simulink model "windEmulatorStep4_WECSim"  (R2025b)
settings: Solver=ode14x  StartTime=0  StopTime=400  FixedStep=Ts  MaxStep=0.01  RelTol=1e-3
values from neighbouring files (symbols this model uses):
  A = 1.0    (= 1)    [initStep4.m]
  absEncoderCountsToRad = 1/2^20*2*pi    (= 5.99211245268e-06)    [initStep4.m]
  acs800CtrlStruct =     [windEmulatorBusDefs.mat]
  acs800DcBusVoltsScaling = 1    [initStep4.m]
  acs800FreqScaling = 1/100    (= 0.01)    [initStep4.m]
  acs800PowerScaling = Gen_PowerScaling    (= 14.9109)    [initStep4.m]
  acs800SignalStruct =     [windEmulatorBusDefs.mat]
  acs800SpeedNomEng = 1500    [initStep4.m]
  acs800SpeedNomFb = 20000    [initStep4.m]
  acs800SpeedScaling = 1500/20000    (= 0.075)    [initStep4.m]
  acs800TempScaling = 1/10    (= 0.1)    [initStep4.m]
  acs800TorqueNomEng = 100    [initStep4.m]
  acs800TorqueNomFb = 10000    [initStep4.m]
  acs800TorqueScaling = acs800TorqueRating/10000    (= 0.008035933)    [initStep4.m]
  acs880CtrlStruct =     [windEmulatorBusDefs.mat]
  acs880FreqScaling = 60/20000    (= 0.003)    [initStep4.m]
  acs880MotorCurrentScaling = 100/10000    (= 0.01)    [initStep4.m]
  acs880MotorVoltsScaling = 1    [initStep4.m]
  acs880PowerScaling = 100*hp2W/10000    (= 7.457)    [initStep4.m]
  acs880RatedTorque = 80.494    [initStep4.m]
  acs880RateLimFalling = -10000    [initStep4.m]
  acs880RateLimRising = 10000    [initStep4.m]
  acs880SetpointLimLower = -0.975*acs880RatedTorque    (= -78.48165)    [initStep4.m]
  acs880SetpointLimUpper = 0.975*acs880RatedTorque    (= 78.48165)    [initStep4.m]
  acs880SignalStruct =     [windEmulatorBusDefs.mat]
  acs880SpeedPILimLo = -0.975*acs880RatedTorque    (= -78.48165)    [initStep4.m]
  acs880SpeedPILimUp = 0.975*acs880RatedTorque    (= 78.48165)    [initStep4.m]
  acs880SpeedScaling = 2000/20000    (= 0.1)    [initStep4.m]
  acs880TorqueFieldbusScale = 10000    [initStep4.m]
  acs880TorqueScaling = acs880RatedTorque/acs880TorqueFieldbusScale    (= 0.0080494)    [initStep4.m]
  acs880TorqueSetpointScaling = 100    [initStep4.m]
  bar2pa = 1e5    (= 100000)    [initStep4.m]
  belowMinPGain = 1/200    (= 0.005)    [initStep4.m]
  ctrlModeTorque = logical(true)    [init.m]    (also in initStep1.m; initStep2.m; initStep3.m; initStep4.m)
  ctrlSignal1 = squeeze(hptoSignalsData.Values.ctrlSignal1.Data)    [postProcessingStep2.m]
  ctrlSignal2 = squeeze(hptoSignalsData.Values.ctrlSignal2.Data)    [postProcessingStep2.m]
  deadBandController = boolean(false)    [initStep4.m]
  deadbandTorqueSlewRate = 300    [initStep4.m]
  Dm_max = 40    [initStep4.m]
  EffMechMax = 0.93    [initStep4.m]
  EffMechMin = 0.79    [initStep4.m]
  excForce_N = squeeze(hptoCtrlData.Values.excForce_N.Data)    [postProcessingStep2.m]
  expCtrlStruct =     [windEmulatorBusDefs.mat]
  FactorEff = psi2pa*cc2m3*(1/rev2rad)    (= 0.00109733470463)    [initStep4.m]
  fromFileSpeedSlewRate = 250    [initStep4.m]
  fromFileTorqueSlewRate = 25    [initStep4.m]
  futekTorqueScale = -1/(2^31)*10/5*100    (= -9.31322574615e-08)    [initStep4.m]
  genMaxTorque = 0.8*ratedTorque    (= 64.3952)    [initStep3.m]    (also in initStep4.m = 78.48165)
  genTorqueCmd_Nm = squeeze(hptoSignalsData.Values.genTorqueCmd_Nm.Data)    [postProcessingStep2.m]
  hbmCtScale = 1/1.5    (= 0.666666666667)    [initStep4.m]
  hbmPowerStruct =     [windEmulatorBusDefs.mat]
  hptoCtrlStruct =     [windEmulatorBusDefs.mat]
  hptoSignalStruct =     [windEmulatorBusDefs.mat]
  invPowerStruct =     [windEmulatorBusDefs.mat]
  lpm2m3ps = 1/m3ps2lpm    (= 1.66666666667e-05)    [initStep4.m]
  minPressureRef_psi = 1000    [initStep4.m]
  minTorqueRef_Nm = (minPressureRef_psi*psi2pa)*(Dm_max*cc2m3*(1/rev2rad))    (= 43.8933881851)    [initStep4.m]
  motorSpeed_rpm = squeeze(acs880SignalsData.Values.motorSpeed_rpm.Data)    [postProcessingStep2.m]
  nPreDrop = 2900    [initStep4.m]
  nPreDropMin = 725    [initStep4.m]
  psi2bar = 1/bar2psi    (= 0.0689475729318)    [initStep4.m]
  radps2rpm = 60/(2*pi)    (= 9.54929658551)    [initStep2.m]    (also in initStep4.m)
  rpm2radps = 2*pi/60    (= 0.10471975512)    [initStep4.m]
  runCounter = squeeze(hptoCtrlData.Values.runCounter.Data)    [postProcessingStep2.m]
  shaftSignalStruct =     [windEmulatorBusDefs.mat]
  sidCtrlStruct =     [windEmulatorBusDefs.mat]
  sidDataCaseCounter = sidData.experimentData.count    [initStep4.m]
  sidDataSpeed_rpm = sidData.experimentData.wShaft_rpm    [initStep4.m]
  sidDataTorque_Nm = sidData.experimentData.torqueShaft_Nm    [initStep4.m]
  sidInfoStruct =     [windEmulatorBusDefs.mat]
  T = 4    [initStep4.m]
  targetOmega = 2000/60*2*pi    (= 209.439510239)    [initStep2.m]    (also in initStep3.m; initStep4.m)
  time = hptoCtrlData.Values.runCounter.Time    [postProcessingStep2.m]
  TorqueLoadMax = 75    [initStep4.m]
  Ts = 1/250    (= 0.004)    [initStep4.m]
undefined symbols (not defined in the file or in its folder): absEncoderCounts, absEncoderPosition_rad, absEncoderSpeed_rpm, absEncoderStatus1, absEncoderStatus2, absEncoderTurns, accVolHP, acs800Torque_Nm, acs800TorqueSetpoint_Nm, acs880SpeedSetpoint_rpm, acs880Torque_Nm, body, constraint, crankLength, ctrlWord, dcBusVoltage_V, DiscIntNeverNeededParam, Dmax, excShaftSpeed_rpm, excShaftTorque_Nm, expType, expTypeEnum, frequency_Hz, fromFileCaseCounter, genPumpFlow_lpm, genShaftSpeed_rpm, genShaftSpeedRef, genSpeedActual, hmOutputShafTorque_Nm, iGainGen, m3persecond2lpm, motorCurrent_A, motorTorque_Nm, motorVoltage_V, offsetLength, pa2psi, pGainGen, pressure_bar, PressureControl, pto, radsec2rpm, ramp, resetHilIntegrator, resetSidIntegrator, rodLength, runHil, runSid, shaftPower_W, sidType, sidTypeEnum, SpeedControl, speedCtrlReset, speedRef_rpm, state, statusWord, stepCounter, temperature, torqueActual_Nm, TorqueInputControl, torqueSetpoint_Nm ... (+1)
libraries: slrealtimeethercatlib x118, fl_lib x81, nesl_utility x45, sh_lib x18, slrealtimeloglib x13, dspstat3 x5, slpidlib x4, simulink_extras x4, cstblocks x3, dspindex x3, WECSim_Lib_Body_Elements x2, simulink x2
(part 4 of 6)

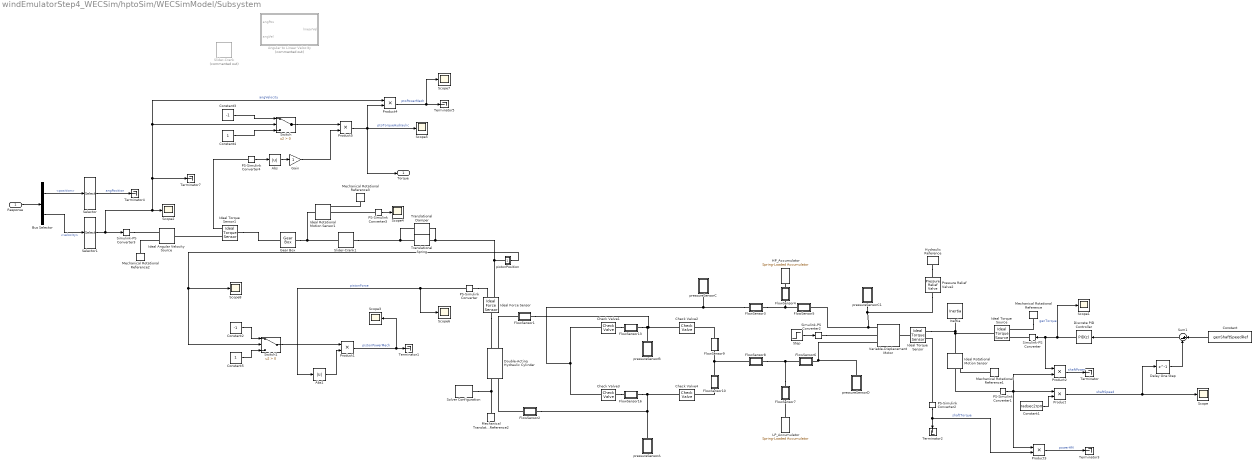
== system windEmulatorStep4_WECSim/hptoSim/WECSimModel/Subsystem ==
  Response : Inport
  Abs : Abs  SaturateOnIntegerOverflow=off
  Abs1 : Abs  SaturateOnIntegerOverflow=off
  Angular to Linear Velocity : Subsystem  Commented=on  AncestorBlock=|
      | WECSim_Lib_PTOSim/Motion Conversion/Rotary to Linear
      | Crank/Angular to Linear
      | Velocity
  Bus Selector : BusSelector  OutputSignals=position,velocity
  Check Valve1 : sh_lib/Valves/Directional Valves/Check Valve  area_max=areaMaxValve m^2  pres_crack=pCrack psi  pres_max=pMaxValve psi  C_d=0.7  A_leak=1e-12 m^2  lam_spec=1  B_lam=0.999  Re_cr=12  dynamic=0  tau=0.1 s  area_init=1e-12 m^2
      settings: InternalSimscapePortConfiguration="{\"Bottom\":[],\"Left\":[{\"id\":\"A\",\"label\":\"A\",\"type\":\"foundation.hydraulic.hydraulic\"}],\"Right\":[{\"id\":\"B\",\"label\":\"B\",\"type\":\"foundation.hydraulic.hydraulic\"}],\"Top\":[]}"
  Check Valve2 : sh_lib/Valves/Directional Valves/Check Valve  area_max=areaMaxValveLP m^2  pres_crack=pCrackLP psi  pres_max=pMaxValveLP psi  C_d=0.7  A_leak=1e-12 m^2  lam_spec=1  B_lam=0.999  Re_cr=12  dynamic=0  tau=0.1 s  area_init=1e-12 m^2
      settings: InternalSimscapePortConfiguration="{\"Bottom\":[],\"Left\":[{\"id\":\"A\",\"label\":\"A\",\"type\":\"foundation.hydraulic.hydraulic\"}],\"Right\":[{\"id\":\"B\",\"label\":\"B\",\"type\":\"foundation.hydraulic.hydraulic\"}],\"Top\":[]}"
  Check Valve3 : sh_lib/Valves/Directional Valves/Check Valve  area_max=areaMaxValve m^2  pres_crack=pCrack psi  pres_max=pMaxValve psi  C_d=0.7  A_leak=1e-12 m^2  lam_spec=1  B_lam=0.999  Re_cr=12  dynamic=0  tau=0.1 s  area_init=1e-12 m^2
      settings: InternalSimscapePortConfiguration="{\"Bottom\":[],\"Left\":[{\"id\":\"A\",\"label\":\"A\",\"type\":\"foundation.hydraulic.hydraulic\"}],\"Right\":[{\"id\":\"B\",\"label\":\"B\",\"type\":\"foundation.hydraulic.hydraulic\"}],\"Top\":[]}"
  Check Valve4 : sh_lib/Valves/Directional Valves/Check Valve  area_max=areaMaxValveLP m^2  pres_crack=pCrackLP psi  pres_max=pMaxValveLP psi  C_d=0.7  A_leak=1e-12 m^2  lam_spec=1  B_lam=0.999  Re_cr=12  dynamic=0  tau=0.1 s  area_init=1e-12 m^2
      settings: InternalSimscapePortConfiguration="{\"Bottom\":[],\"Left\":[{\"id\":\"A\",\"label\":\"A\",\"type\":\"foundation.hydraulic.hydraulic\"}],\"Right\":[{\"id\":\"B\",\"label\":\"B\",\"type\":\"foundation.hydraulic.hydraulic\"}],\"Top\":[]}"
  Constant : Constant  Value=genShaftSpeedRef
  Constant1 : Constant  Value=radsec2rpm
  Constant2 : Constant  Value=-1
  Constant3 : Constant  Value=-1
  Constant4 : Constant
  Constant5 : Constant
  Delay One Step : Delay  DelayLength=1
  Discrete PID Controller : slpidlib/PID Controller  Controller=PID  Form=Parallel  TimeDomain=Discrete-time  UseExternalTs=off  SampleTime=-1  IntegratorMethod=Forward Euler  FilterMethod=Forward Euler  ControllerParametersSource=internal  P=pGainGen  I=iGainGen  UseKiTs=off  D=0  UseExternalDerivativeSource=off  N=100  UseFilter=off  TunerSelectOption=Transfer Function Based (PID Tuner App)  InitialConditionSource=internal  InitialConditionForIntegrator=0  InitialConditionForFilter=0  DifferentiatorICPrevScaledInput=0  ExternalReset=none  TrackingMode=off  Kt=1  LimitOutput=off  SatLimitsSource=internal  UpperSaturationLimit=inf  LowerSaturationLimit=-inf  LinearizeAsGain=off  AntiWindupMode=none  Kb=1  LimitIntegrator=off  UpperIntegratorSaturationLimit=inf  LowerIntegratorSaturationLimit=-inf  POutMin=[]  POutMax=[]  IOutMin=[]  IOutMax=[]  DOutMin=[]  DOutMax=[]  NOutMin=[]  NOutMax=[]  SumOutMin=[]  SumOutMax=[]  SaturationOutMin=[]  SaturationOutMax=[]  PParamMin=[]  PParamMax=[]  IParamMin=[]  IParamMax=[]  DParamMin=[]  DParamMax=[]  NParamMin=[]  NParamMax=[]  KbParamMin=[]  KbParamMax=[]  KtParamMin=[]  KtParamMax=[]  KbOutMin=[]  KbOutMax=[]  KtOutMin=[]  KtOutMax=[]  IntegratorOutMin=[]  IntegratorOutMax=[]  FilterOutMin=[]  FilterOutMax=[]  SumI1OutMin=[]  SumI1OutMax=[]  SumI2OutMin=[]  SumI2OutMax=[]  SumI3OutMin=[]  SumI3OutMax=[]  SumI4OutMin=[]  SumI4OutMax=[]  SumDOutMin=[]  SumDOutMax=[]  DifferentiatorOutMin=[]  DifferentiatorOutMax=[]  FilterDiffOutCoefMin=[]  FilterDiffOutCoefMax=[]  ReciprocalOutMin=[]  ReciprocalOutMax=[]  SumDenOutMin=[]  SumDenOutMax=[]  SumNumOutMin=[]  SumNumOutMax=[]  DivideOutMin=[]  DivideOutMax=[]  UdiffTsProdOutMin=[]  UdiffTsProdOutMax=[]  NTsProdOutMin=[]  NTsProdOutMax=[]  UintegralTsProdOutMin=[]  UintegralTsProdOutMax=[]  UngainTsProdOutMin=[]  UngainTsProdOutMax=[]  ClampingZeroOutDataTypeStr=Inherit: Inherit via back propagation  ClampingZeroOutMin=[]  ClampingZeroOutMax=[]  FilterDenConstantOutDataTypeStr=Inherit: Inherit via back propagation  FilterDenConstantOutMin=[]  FilterDenConstantOutMax=[]  PCopyOutDataTypeStr=Inherit: Inherit via back propagation  PCopyOutMin=[]  PCopyOutMax=[]  NCopyOutDataTypeStr=Inherit: Inherit via back propagation  NCopyOutMin=[]  NCopyOutMax=[]  IntegratorContinuousStateAttributes=''  IntegratorStateMustResolveToSignalObject=off  IntegratorRTWStateStorageClass=Auto  FilterContinuousStateAttributes=''  FilterStateMustResolveToSignalObject=off  FilterRTWStateStorageClass=Auto  ParallelPVariant=InternalParameters  IdealPVariant=Disabled  IVariant=InternalParameters  DVariant=InternalParameters  IntegratorVariant=Discrete  SatVariant=Disabled  AWVariant=Passthrough  PCopyVariant=Disabled  TRVariant=Disabled  FdbkBlocksVariant=Forward  IdealPFdbkVariant=Disabled  SatFdbkVariant=Disabled  DerivativeFilterVariant=Differentiator  NVariant=Passthrough  NCopyVariant=Disabled_SignalSpec  FilterICVariant=InternalICsDifferentiator  IntegratorICVariant=InternalICs  ExternalResetVariant=Disabled  TRSumVariant=Passthrough  SumFdbkVariant=Disabled  SumVariant=Sum_PID  TsampFilterVariant=InternalTs  TsampNgainVariant=Passthrough  TsampIntegralVariant=Disabled_SignalSpec  ExternalSaturationOutDataTypeStr=Inherit: Same as second input  DerivativeSourceVariant=ErrorSignal  PreIntVariant=InternalPreInt
      settings: LibrarySourceBlock=simulink/Discrete/Discrete PID Controller
  Double-Acting Hydraulic Cylinder : sh_lib/Hydraulic Cylinders/Double-Acting Hydraulic Cylinder  area_A=areaHC m^2  area_B=areaHC m^2  stroke=strokePiston m  dead_vol_A=deadVolume m^3  dead_vol_B=deadVolume m^3  k_sh=1.4  or=sh.cylinders.enum.MechOrientationTranslational.Positive  stiff=1e6 N/m  D=150 N*s/m  hardstop_model=1  transition=0.1 mm  displacement_spec=foundation.enum.DisplacementSpec.Calculate  init_pos=pistonInitialPos m  init_pressure_A=0 Pa  init_pressure_B=0 Pa
      settings: InternalSimscapePortConfiguration="{\"Bottom\":[],\"Left\":[{\"id\":\"C\",\"label\":\"C\",\"type\":\"foundation.mechanical.translational.translational\"},{\"id\":\"A\",\"label\":\"A\",\"type\":\"foundation.hydraulic.hydraulic\"}],\"Right\":[{\"id\":\"R\",\"label\":\"R\",\"type\":\"foundation.mechanical.translational.translational\"},{\"id\":\"B\",\"label\":\"B\",\"type\":\"foundation.hydraulic.hydraulic\"}],\"Top\":[]}"
  FlowSensor1 : Subsystem
  FlowSensor10 : Subsystem
  FlowSensor13 : Subsystem
  FlowSensor16 : Subsystem
  FlowSensor2 : Subsystem
  FlowSensor3 : Subsystem
  FlowSensor4 : Subsystem
  FlowSensor5 : Subsystem
  FlowSensor6 : Subsystem
  FlowSensor7 : Subsystem
  FlowSensor8 : Subsystem
  FlowSensor9 : Subsystem
  Gain : Gain
  Gear Box : fl_lib/Mechanical/Mechanisms/Gear Box  ratio=1/5  t_in_specify=off  t_in_priority=None  t_in=0 N*m  t_in_nominal_specify=off  t_in_nominal_value=1  t_in_nominal_unit=N*m  t_out_specify=off  t_out_priority=None  t_out=0 N*m  t_out_nominal_specify=off  t_out_nominal_value=1  t_out_nominal_unit=N*m
  HP_Accumulator : sh_lib/Accumulators/Spring-Loaded Accumulator  capacity=accVolHP l  pr_preload=pPreLoadHP psi  pr_max=pMaxAccHP psi  stiff_coeff=1e10 Pa/m^3  penetr_coeff=1e10 Pa*s/m^6  flow_rate_specify=off  flow_rate_priority=None  flow_rate=5e-3 m^3/s  flow_rate_nominal_specify=off  flow_rate_nominal_value=1  flow_rate_nominal_unit=m^3/s  fluid_volume_specify=off  fluid_volume_priority=High  fluid_volume=accVolHP*0.01 l  fluid_volume_nominal_specify=off  fluid_volume_nominal_value=1  fluid_volume_nominal_unit=m^3  fluid_pressure_specify=off  fluid_pressure_priority=None  fluid_pressure=1.01325e5 Pa  fluid_pressure_nominal_specify=off  fluid_pressure_nominal_value=1  fluid_pressure_nominal_unit=Pa
      settings: InternalSimscapePortConfiguration="{\"Bottom\":[],\"Left\":[],\"Right\":[{\"id\":\"A\",\"label\":\"A\",\"type\":\"foundation.hydraulic.hydraulic\"}],\"Top\":[]}"
  Hydraulic Reference : fl_lib/Hydraulic/Hydraulic Elements/Hydraulic Reference
  Ideal Angular Velocity Source : fl_lib/Mechanical/Mechanical Sources/Ideal Angular Velocity Source
  Ideal Force Sensor : fl_lib/Mechanical/Mechanical Sensors/Ideal Force Sensor
  Ideal Rotational Motion Sensor : fl_lib/Mechanical/Mechanical Sensors/Ideal Rotational Motion Sensor  reference=foundation.enum.MeasurementReference.difference  acceleration_port=false  velocity_port=true  position_port=true  wrap_angle=false  offset=0 rad
  Ideal Rotational Motion Sensor1 : fl_lib/Mechanical/Mechanical Sensors/Ideal Rotational Motion Sensor  reference=foundation.enum.MeasurementReference.difference  acceleration_port=false  velocity_port=true  position_port=true  wrap_angle=false  offset=0 rad
  Ideal Torque Sensor : fl_lib/Mechanical/Mechanical Sensors/Ideal Torque Sensor
  Ideal Torque Sensor1 : fl_lib/Mechanical/Mechanical Sensors/Ideal Torque Sensor
  Ideal Torque Source : fl_lib/Mechanical/Mechanical Sources/Ideal Torque Source
  Inertia : fl_lib/Mechanical/Rotational Elements/Inertia  inertia=50 kg*m^2  num_ports=foundation.enum.numPorts2.one  w_specify=off  w_priority=High  w=genShaftSpeedRef rpm  w_nominal_specify=off  w_nominal_value=1  w_nominal_unit=rad/s  t_specify=off  t_priority=None  t=0 N*m  t_nominal_specify=off  t_nominal_value=1  t_nominal_unit=N*m
  LP_Accumulator : sh_lib/Accumulators/Spring-Loaded Accumulator  capacity=accVolLP l  pr_preload=pPreLoadLP psi  pr_max=pMaxAccLP psi  stiff_coeff=1e10 Pa/m^3  penetr_coeff=1e10 Pa*s/m^6  flow_rate_specify=off  flow_rate_priority=None  flow_rate=5e-3 m^3/s  flow_rate_nominal_specify=off  flow_rate_nominal_value=1  flow_rate_nominal_unit=m^3/s  fluid_volume_specify=off  fluid_volume_priority=High  fluid_volume=accVolLP m^3  fluid_volume_nominal_specify=off  fluid_volume_nominal_value=1  fluid_volume_nominal_unit=m^3  fluid_pressure_specify=off  fluid_pressure_priority=None  fluid_pressure=1.01325e5 Pa  fluid_pressure_nominal_specify=off  fluid_pressure_nominal_value=1  fluid_pressure_nominal_unit=Pa
      settings: InternalSimscapePortConfiguration="{\"Bottom\":[],\"Left\":[],\"Right\":[{\"id\":\"A\",\"label\":\"A\",\"type\":\"foundation.hydraulic.hydraulic\"}],\"Top\":[]}"
  Mechanical Rotational Reference{,1..3} (4 alike) : fl_lib/Mechanical/Rotational Elements/Mechanical Rotational Reference
  Mechanical Translational Reference2 : fl_lib/Mechanical/Translational Elements/Mechanical Translational Reference
  PS-Simulink Converter{,1..4} (5 alike) : nesl_utility/PS-Simulink Converter  PhysicalDomain=network_engine_domain  SubClassName=ps_output  LeftPortType=input  RightPortType=output  PseudoPeriodic=off  Frequencies=[]  VectorFormat=inherit  Unit=inherit  AffineConversion=off
  Pressure Relief Valve2 : sh_lib/Valves/Pressure Control Valves/Pressure Relief Valve  valve_area_spec=1  p_diff_TLU=[30.15e5 : 15e3 : 31.35e5] Pa  area_TLU=[1 : 1 : 9] .* 1e-5 m^2  area_max=2.2e-4 m^2  pres_set=4900 psi  reg_range=10 psi  C_d=0.7  A_leak=1e-12 m^2  lam_spec=1  B_lam=0.999  Re_cr=12  dynamic=0  tau=0.1 s  area_init=1e-12 m^2
      settings: InternalSimscapePortConfiguration="{\"Bottom\":[],\"Left\":[{\"id\":\"A\",\"label\":\"A\",\"type\":\"foundation.hydraulic.hydraulic\"}],\"Right\":[{\"id\":\"B\",\"label\":\"B\",\"type\":\"foundation.hydraulic.hydraulic\"}],\"Top\":[]}"
  Product{,1..5} (6 alike) : Product
  Scope{,1..8} (9 alike) : Scope
      Scope settings: ActiveDisplayYMinimum=1738.7756957222209  ActiveDisplayYMaximum=1946.7249509603892
      Scope1 settings: ActiveDisplayYMinimum=-94.135566599802871  ActiveDisplayYMaximum=67.441074091156352
      Scope2 settings: ActiveDisplayYMinimum=-0.31429832837768534  ActiveDisplayYMaximum=0.30729177387363948  DataLoggingVariableName=ScopeData2
      Scope3 settings: ActiveDisplayYMinimum=-0.10262196705005888  ActiveDisplayYMaximum=0.14966467708972742  DataLoggingVariableName=ScopeData8
      Scope4 settings: ActiveDisplayYMinimum=-3.77179135660224  ActiveDisplayYMaximum=3.7759988528286708  DataLoggingVariableName=ScopeData9
      Scope5 settings: ActiveDisplayYMinimum=-1.4215512241951279E+7  ActiveDisplayYMaximum=1.4218962302598771E+7  DataLoggingVariableName=ScopeData10
      Scope6 settings: ActiveDisplayYMinimum=-1.9695787856257146E+6  ActiveDisplayYMaximum=1.571747168448562E+6  DataLoggingVariableName=ScopeData11
      Scope7 settings: ActiveDisplayYMinimum=-1.8232047357809118E+6  ActiveDisplayYMaximum=202578.3039756568  DataLoggingVariableName=ScopeData12
      Scope8 settings: DataLoggingVariableName=ScopeData13
  Selector : Selector  InputPortWidth=6  IndexOptions=Index vector (dialog)  Indices=5  OutputSizes=1
  Selector1 : Selector  InputPortWidth=6  IndexOptions=Index vector (dialog)  Indices=5  OutputSizes=1
  Simulink-PS Converter : nesl_utility/Simulink-PS Converter  PhysicalDomain=network_engine_domain  SubClassName=ps_input  LeftPortType=input  RightPortType=output  PseudoPeriodic=off  Frequencies=[]  NoiseDistribution=none  NoiseParameters=[]  Unit=1  AffineConversion=off  FilteringAndDerivatives=provide  SimscapeFilterOrder=1  InputFilterTimeConstant=0.001  UdotUserProvided=0
  Simulink-PS Converter2 : nesl_utility/Simulink-PS Converter  PhysicalDomain=network_engine_domain  SubClassName=ps_input  LeftPortType=input  RightPortType=output  PseudoPeriodic=off  Frequencies=[]  NoiseDistribution=none  NoiseParameters=[]  Unit=1  AffineConversion=off  FilteringAndDerivatives=provide  SimscapeFilterOrder=1  InputFilterTimeConstant=0.001  UdotUserProvided=0
  Simulink-PS Converter3 : nesl_utility/Simulink-PS Converter  PhysicalDomain=network_engine_domain  SubClassName=ps_input  LeftPortType=input  RightPortType=output  PseudoPeriodic=off  Frequencies=[]  NoiseDistribution=none  NoiseParameters=[]  Unit=1  AffineConversion=off  FilteringAndDerivatives=filter  SimscapeFilterOrder=1  InputFilterTimeConstant=0.001  UdotUserProvided=0
  Slider-Crank : fl_lib/Mechanical/Mechanisms/Slider-Crank  Commented=on  crank=crankLength m  rod=rodLength m  inertia=0.01 kg*m^2  k=1e6 N/m  b=1e3 N*s/m  theta_specify=off  theta_priority=High  theta=pi / 2 rad  theta_nominal_specify=off  theta_nominal_value=1  theta_nominal_unit=rad  w_specify=off  w_priority=High  w=0 rad/s  w_nominal_specify=off  w_nominal_value=1  w_nominal_unit=rad/s
      settings: InternalSimscapePortConfiguration="{\"Bottom\":[],\"Left\":[{\"id\":\"C\",\"label\":\"C\",\"type\":\"foundation.mechanical.rotational.rotational\"}],\"Right\":[{\"id\":\"S\",\"label\":\"S\",\"type\":\"foundation.mechanical.translational.translational\"}],\"Top\":[]}"
  Slider-Crank1 : fl_lib/Mechanical/Mechanisms/Slider-Crank  crank=2 m  rod=4 m  inertia=0.01 kg*m^2  k=1e6 N/m  b=1e3 N*s/m  theta_specify=off  theta_priority=High  theta=pi / 2 rad  theta_nominal_specify=off  theta_nominal_value=1  theta_nominal_unit=rad  w_specify=off  w_priority=High  w=0 rad/s  w_nominal_specify=off  w_nominal_value=1  w_nominal_unit=rad/s
      settings: InternalSimscapePortConfiguration="{\"Bottom\":[],\"Left\":[{\"id\":\"C\",\"label\":\"C\",\"type\":\"foundation.mechanical.rotational.rotational\"}],\"Right\":[{\"id\":\"S\",\"label\":\"S\",\"type\":\"foundation.mechanical.translational.translational\"}],\"Top\":[]}"
  Solver Configuration : nesl_utility/Solver Configuration  PhysicalDomain=network_engine_domain  SubClassName=solver  LeftPortType=input  RightPortType=generic  Tones=[]  Harmonics=[]  SimulateNoise=off  Profile=off  UseLocalSampling=off  EnableSwitchedLinearOptims=on  FrequencyDomain=off  UseCCode=off  RelTol=0.001  AbsTol=0.001  MinStep=1e-09  ToWorkspace=off  RevertToSquareIcSolve=off  NumHomotopyIterations=100  PhasorMode=off  PhasorModeNumHarmonics=1  ConsistencySolver=NEWTON_XTOL_AFTER_FTOL  IndexReductionMethod=DerivativeReplacement  DoDC=off  ResidualTolerance=1e-09  ConsistencyTolSource=GLOBAL  ConsistencyAbsTol=0.001  ConsistencyRelTol=0.001  ConsistencyTolFactor=0.001  UseLocalSolver=off  LocalSolverChoice=NE_BACKWARD_EULER_ADVANCER  ResolveIndetEquations=on  FunctionEvalNumThread=1  LocalSolverSampleTime=0.001  DoFixedCost=off  MaxNonlinIter=3  MaxModeIter=2  ComputeImpulses=off  ImpulseIterations=2  LinearAlgebra=auto  LinearAlgebraNumThread=0  EquationFormulation=NE_TIME_EF  DelaysMemoryBudget=1024  AutomaticFiltering=on  FilteringTimeConstant=0.001  PartitionStorageMethod=AS_NEEDED  PartitionMemoryBudget=1024  PartitionMethod=ROBUST  MultibodyUseLocalSolver=off  MultibodyLocalSolverChoice=ODE1  MultibodyLocalSolverSampleTime=0.001
  Step : Step  Time=100  Before=0.0075  After=0.0075  SampleTime=0
  Sum1 : Sum  Inputs=|+-
  Switch : Switch  Criteria=u2 > Threshold  SaturateOnIntegerOverflow=off  InputSameDT=off
  Switch1 : Switch  Criteria=u2 > Threshold  SaturateOnIntegerOverflow=off  InputSameDT=off
  Terminator{,1..5,7} (7 alike) : Terminator
  Translational Damper : sdl_lib/Couplings & Drives/Springs & Dampers/Translational Damper  D=14000 N*s/m  thermal_port=simscape.enum.thermaleffects.omit  thermal_mass=50 kJ/K  temperature_specify=off  temperature_priority=High  temperature=300 K  temperature_nominal_specify=off  temperature_nominal_value=1  temperature_nominal_unit=K
  Translational Spring : fl_lib/Mechanical/Translational Elements/Translational Spring  spr_rate=1e7 N/m  v_specify=off  v_priority=None  v=0 m/s  v_nominal_specify=off  v_nominal_value=1  v_nominal_unit=m/s  f_specify=off  f_priority=None  f=0 N  f_nominal_specify=off  f_nominal_value=1  f_nominal_unit=N  x_specify=off  x_priority=High  x=0 m  x_nominal_specify=off  x_nominal_value=1  x_nominal_unit=m
  Variable-Displacement Motor : sh_lib/Pumps and Motors/Variable-Displacement Motor  mdl_type=2  stroke_max=0.005 m  D_max=Dmax cm^3/rev  cntrl_mem_tab="[-.0075, 0,  .0075] m"  displ_tab=[-Dmax, 0, Dmax] cm^3/rev  interp_method=1  extrap_method=1  loss_spec=1  w_nominal=shaftSpeedNominal rpm  pr_nominal=pressureNom psi  visc_nominal=kinematicVisNom cSt  dens_nominal=fluidDensityNom kg/m^3  efficiency_vol=0.92  no_load_torque=noLoadTorque N*m  torque_pressure_coeff=frictionTorqueVsPressure N*m/Pa  p_diff_eff_TLU=[100000, 1000000, 2000000] Pa  omega_eff_TLU=[25, 50, 100, 200, 300, 400] rad/s  displacement_eff_TLU=[-30, -19, 19, 30] cm^3/rev  vol_eff_TLU=repmat([.816, .908, .954, .977, .981, .984; .325, .663, .831, .916, .925, .946; .137, .568, .78, .892, .893, .91], 1, 1, 4)  mech_eff_TLU=repmat([.996, .996, .996, .996, .996, .996; .988, .989, .989, .989, .989, .99; .981, .981, .982, .982, .983, .984], 1, 1, 4)  p_diff_loss_TLU=[100000, 1000000, 2000000] Pa  omega_loss_TLU=[25, 50, 100, 200, 300, 400] rad/s  displacement_loss_TLU=[-30, -19, 19, 30] cm^3/rev  vol_loss_TLU=repmat([.0282, .0253, .0241, .0235, .0291, .0325; .2596, .1271, .1017, .0917, .1216, .1142; .7874, .1901, .141, .1211, .1797, .1978] * 1e-3, 1, 1, 4) m^3/s  mech_loss_TLU=repmat([.002, .002, .002, .002, .002, .002; .06, .055, .055, .055, .055, .05; .19, .19, .18, .18, .17, .16], 1, 1, 4) N*m  pressure_threshold=1e5 Pa  omega_threshold=10 rad/s  displacement_threshold=0.5 cm^3/rev  octant_check=0  pressure_check=0  min_valid_pressure=0 Pa  vol_eff_min=1e-3  vol_eff_max=1  mech_eff_min=1e-3  mech_eff_max=1
      settings: InternalSimscapePortConfiguration="{\"Bottom\":[],\"Left\":[{\"id\":\"A\",\"label\":\"A\",\"type\":\"foundation.hydraulic.hydraulic\"},{\"id\":\"C\",\"label\":\"C\",\"type\":\"input\"},{\"id\":\"B\",\"label\":\"B\",\"type\":\"foundation.hydraulic.hydraulic\"}],\"Right\":[{\"id\":\"S\",\"label\":\"S\",\"type\":\"foundation.mechanical.rotational.rotational\"}],\"Top\":[]}"
  pistonPosition : Subsystem
  pressureSensorA : Subsystem
  pressureSensorB : Subsystem
  pressureSensorC : Subsystem
  pressureSensorC1 : Subsystem
  pressureSensorD : Subsystem
  Torque : Outport
  wires:
  PS-Simulink Converter2/1 -> Product3/2, Terminator2/1  "shaftTorque"
  Constant/1 -> Sum1/1
  PS-Simulink Converter1/1 -> Product2/2, Product3/1, Product/1
  Sum1/1 -> Discrete PID Controller/1
  Product1/1 -> Scope3/1, Terminator1/1  "pistonPowerMech"
  Product2/1 -> Terminator/1  "shaftPower"
  Product3/1 -> Terminator3/1  "powerHM"
  PS-Simulink Converter/1 -> Scope6/1, Abs1/1  "pistonForce"
  Step/1 -> Simulink-PS Converter2/1
  Discrete PID Controller/1 -> Product2/1, Simulink-PS Converter/1, Scope1/1  "genTorque"
  Product/1 -> Delay One Step/1, Scope/1  "shaftSpeed"
  Constant1/1 -> Product/2
  Response/1 -> Bus Selector/1
  Bus Selector/1 -> Selector/1  "<position>"
  Selector/1 -> Terminator4/1  "angPosition"
  Bus Selector/2 -> Selector1/1  "<velocity>"
  Selector1/1 -> Product4/1, Switch/2, Terminator7/1, Scope2/1, Simulink-PS Converter3/1  "angVelocity"
  Delay One Step/1 -> Sum1/2
  PS-Simulink Converter3/1 -> Scope4/1
  PS-Simulink Converter4/1 -> Abs/1
  Product4/1 -> Scope7/1, Terminator5/1  "ptoPowerMech"
  Abs/1 -> Gain/1
  Constant3/1 -> Switch/1
  Constant4/1 -> Switch/3
  Switch/1 -> Product5/1
  Gain/1 -> Product5/2
  Product5/1 -> Torque/1, Product4/2, Scope5/1  "ptoTorqueHydraulic"
  Switch1/1 -> Product1/1
  pistonPosition/1(Out1) -> Switch1/2, Scope8/1
  Constant2/1 -> Switch1/1
  Constant5/1 -> Switch1/3
  Abs1/1 -> Product1/2
  connections:
  Check Valve4/RConn1 -- FlowSensor16/LConn1 -- FlowSensor2/RConn1 -- pressureSensorA/LConn1
  FlowSensor9/LConn1 -- FlowSensor8/RConn1 -- FlowSensor10/LConn1
  FlowSensor13/LConn1 -- FlowSensor1/RConn1 -- Check Valve2/RConn1 -- pressureSensorB/LConn1
  pressureSensorC1/LConn1 -- Variable-Displacement Motor/LConn1 -- FlowSensor5/RConn1 -- Pressure Relief Valve2/LConn1
  FlowSensor4/LConn1 -- FlowSensor5/LConn1 -- FlowSensor3/RConn1
  Inertia/LConn1 -- Ideal Rotational Motion Sensor/LConn1 -- Ideal Torque Source/LConn1 -- Ideal Torque Sensor/RConn1
  pressureSensorD/LConn1 -- FlowSensor6/LConn1 -- Variable-Displacement Motor/LConn3
  pistonPosition/LConn1 -- Translational Damper/RConn1 -- Translational Spring/RConn1 -- Ideal Force Sensor/RConn1
  FlowSensor7/LConn1 -- FlowSensor6/RConn1 -- FlowSensor8/LConn1
  FlowSensor3/LConn1 -- Check Valve3/RConn1 -- Check Valve1/RConn1 -- pressureSensorC/LConn1
  Solver Configuration/RConn1 -- Mechanical Translational Reference2/LConn1 -- Double-Acting Hydraulic Cylinder/LConn1
  FlowSensor10/RConn1 -- Check Valve4/LConn1
  FlowSensor9/RConn1 -- Check Valve2/LConn1
  Check Valve1/LConn1 -- FlowSensor13/RConn1
  Hydraulic Reference/LConn1 -- Pressure Relief Valve2/RConn1
  PS-Simulink Converter/LConn1 -- Ideal Force Sensor/RConn2
  Simulink-PS Converter/RConn1 -- Ideal Torque Source/RConn1
  Mechanical Rotational Reference1/LConn1 -- Ideal Rotational Motion Sensor/RConn1
  FlowSensor2/LConn1 -- Double-Acting Hydraulic Cylinder/LConn2
  Simulink-PS Converter2/RConn1 -- Variable-Displacement Motor/LConn2
  FlowSensor1/LConn1 -- Double-Acting Hydraulic Cylinder/RConn2
  FlowSensor4/RConn1 -- HP_Accumulator/RConn1
  Ideal Torque Sensor/LConn1 -- Variable-Displacement Motor/RConn1
  PS-Simulink Converter1/LConn1 -- Ideal Rotational Motion Sensor/RConn2
  LP_Accumulator/RConn1 -- FlowSensor7/RConn1
  Ideal Force Sensor/LConn1 -- Double-Acting Hydraulic Cylinder/RConn1
  PS-Simulink Converter2/LConn1 -- Ideal Torque Sensor/RConn2
  Mechanical Rotational Reference/LConn1 -- Ideal Torque Source/RConn2
  Check Valve3/LConn1 -- FlowSensor16/RConn1
  Simulink-PS Converter3/RConn1 -- Ideal Angular Velocity Source/RConn1
  Gear Box/RConn1 -- Ideal Rotational Motion Sensor1/LConn1 -- Slider-Crank1/LConn1
  Mechanical Rotational Reference2/LConn1 -- Ideal Angular Velocity Source/RConn2
  Mechanical Rotational Reference3/LConn1 -- Ideal Rotational Motion Sensor1/RConn1
  PS-Simulink Converter3/LConn1 -- Ideal Rotational Motion Sensor1/RConn2
  Slider-Crank1/RConn1 -- Translational Damper/LConn1 -- Translational Spring/LConn1
  Ideal Torque Sensor1/LConn1 -- Gear Box/LConn1
  Ideal Torque Sensor1/RConn1 -- Ideal Angular Velocity Source/LConn1
  PS-Simulink Converter4/LConn1 -- Ideal Torque Sensor1/RConn2

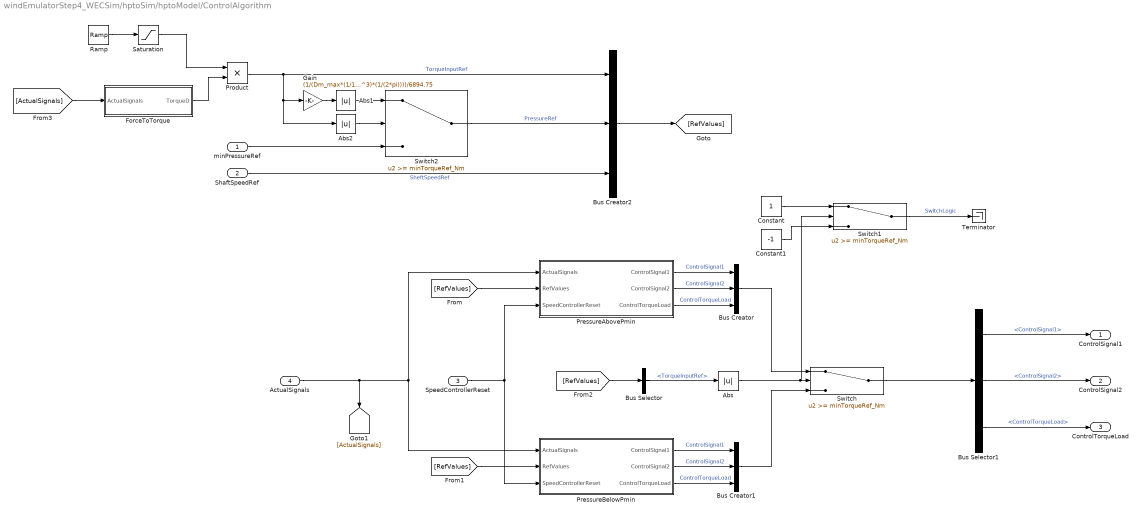
== system windEmulatorStep4_WECSim/hptoSim/hptoModel/ControlAlgorithm ==
  minPressureRef : Inport
  ShaftSpeedRef : Inport  Port=2
  SpeedControllerReset : Inport  Port=3
  ActualSignals : Inport  Port=4
  Abs : Abs  SaturateOnIntegerOverflow=off
  Abs1 : Abs  SaturateOnIntegerOverflow=off
  Abs2 : Abs  SaturateOnIntegerOverflow=off
  Bus Creator : BusCreator  Inputs=3
  Bus Creator1 : BusCreator  Inputs=3
  Bus Creator2 : BusCreator  Inputs=3
  Bus Selector : BusSelector  OutputSignals=TorqueInputRef
  Bus Selector1 : BusSelector  OutputSignals=ControlSignal1,ControlSignal2,ControlTorqueLoad
  Constant : Constant
  Constant1 : Constant  Value=-1
  ForceToTorque : Subsystem
  Gain : Gain  Gain=(1/(Dm_max*(1/100^3)*(1/(2*pi))))/6894.75
  PressureAbovePmin : Subsystem
  PressureBelowPmin : Subsystem
  Product : Product
  Ramp : simulink/Sources/Ramp  slope=1/10  start=10  InitialOutput=0
  Saturation : Saturate  UpperLimit=1  LowerLimit=0
  Switch : Switch  Threshold=minTorqueRef_Nm  SaturateOnIntegerOverflow=off  InputSameDT=off
  Switch1 : Switch  Threshold=minTorqueRef_Nm  SaturateOnIntegerOverflow=off  InputSameDT=off
  Switch2 : Switch  Threshold=minTorqueRef_Nm  SaturateOnIntegerOverflow=off  InputSameDT=off
  Terminator : Terminator
  ControlSignal1 : Outport
  ControlSignal2 : Outport  Port=2
  ControlTorqueLoad : Outport  Port=3
  wires:
  ActualSignals/1 -> [ActualSignals], PressureAbovePmin/1(ActualSignals), PressureBelowPmin/1(ActualSignals)
  PressureAbovePmin/1(ControlSignal1) -> Bus Creator/1  "ControlSignal1"
  PressureAbovePmin/2(ControlSignal2) -> Bus Creator/2  "ControlSignal2"
  PressureAbovePmin/3(ControlTorqueLoad) -> Bus Creator/3  "ControlTorqueLoad"
  Bus Creator/1 -> Switch/1
  PressureBelowPmin/1(ControlSignal1) -> Bus Creator1/1  "ControlSignal1"
  PressureBelowPmin/2(ControlSignal2) -> Bus Creator1/2  "ControlSignal2"
  PressureBelowPmin/3(ControlTorqueLoad) -> Bus Creator1/3  "ControlTorqueLoad"
  Bus Creator1/1 -> Switch/3
  Bus Selector1/1 -> ControlSignal1/1  "<ControlSignal1>"
  Bus Selector1/2 -> ControlSignal2/1  "<ControlSignal2>"
  Bus Selector1/3 -> ControlTorqueLoad/1  "<ControlTorqueLoad>"
  Product/1 -> Bus Creator2/1, Abs2/1, Gain/1  "TorqueInputRef"
  ShaftSpeedRef/1 -> Bus Creator2/3  "SheftSpeedRef"
  Bus Creator2/1 -> [RefValues]
  [RefValues] -> PressureAbovePmin/2(RefValues)
  [RefValues] -> PressureBelowPmin/2(RefValues)
  [RefValues] -> Bus Selector/1
  Bus Selector/1 -> Abs/1  "<TorqueInputRef>"
  Abs/1 -> Switch1/2, Switch/2
  Constant/1 -> Switch1/1
  Constant1/1 -> Switch1/3
  Switch1/1 -> Terminator/1  "SwitchLogic"
  Gain/1 -> Abs1/1
  Abs1/1 -> Switch2/1
  minPressureRef/1 -> Switch2/3
  Abs2/1 -> Switch2/2
  Switch2/1 -> Bus Creator2/2  "PressureRef"
  Saturation/1 -> Product/1
  Ramp/1 -> Saturation/1
  [ActualSignals] -> ForceToTorque/1(ActualSignals)
  ForceToTorque/1(TorqueD) -> Product/2
  Switch/1 -> Bus Selector1/1
  SpeedControllerReset/1 -> PressureAbovePmin/3(SpeedControllerReset), PressureBelowPmin/3(SpeedControllerReset)

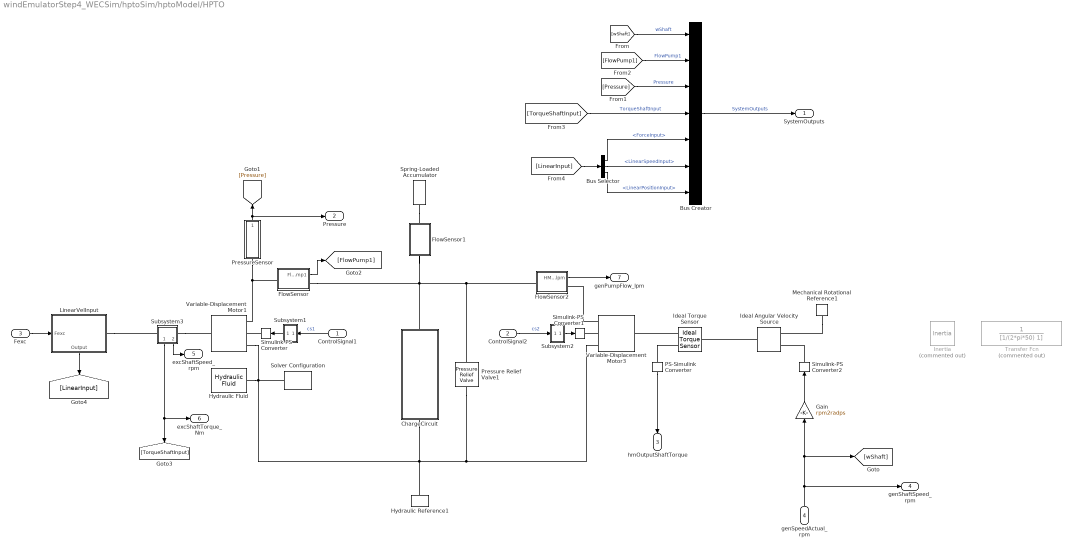
== system windEmulatorStep4_WECSim/hptoSim/hptoModel/HPTO ==
  ControlSignal1 : Inport
  ControlSignal2 : Inport  Port=2
  Fexc : Inport  Port=3
  genSpeedActual_rpm : Inport  Port=4
  Bus Creator : BusCreator  Inputs=7
  Bus Selector : BusSelector  OutputSignals=ForceInput,LinearSpeedInput,LinearPositionInput
  ChargeCircuit : Subsystem
  FlowSensor : Subsystem
  FlowSensor1 : Subsystem
  FlowSensor2 : Subsystem
  Gain : Gain  Gain=rpm2radps
  Hydraulic Fluid : sh_lib/Hydraulic Utilities/Hydraulic Fluid  SelFluid=1  SysTemp=60  TrapAir=0.005  ViscDerFactor=1  range_error=1  suppress_warning=false
  Hydraulic Reference1 : fl_lib/Hydraulic/Hydraulic Elements/Hydraulic Reference
  Ideal Angular Velocity Source : fl_lib/Mechanical/Mechanical Sources/Ideal Angular Velocity Source
  Ideal Torque Sensor : fl_lib/Mechanical/Mechanical Sensors/Ideal Torque Sensor
  Inertia : fl_lib/Mechanical/Rotational Elements/Inertia  Commented=on  inertia=genShaftInertia_kgm2 kg*m^2  num_ports=foundation.enum.numPorts2.one  w_specify=off  w_priority=High  w=0 rad/s  w_nominal_specify=off  w_nominal_value=1  w_nominal_unit=rad/s  t_specify=off  t_priority=None  t=0 N*m  t_nominal_specify=off  t_nominal_value=1  t_nominal_unit=N*m
  LinearVelInput : Subsystem
      settings: PortSchema="{\"entries\":[{\"content\":{\"sides\":[{\"content\":{\"connectorIds\":[\"LConn1\"]},\"type\":\"ConnectorPlacement.EquallySpacedRectSide\",\"uuid\":\"4859a0f7-9f9b-474b-bb49-bd256c408622\"},{\"content\":{\"connectorIds\":[\"In1\"],\"side\":\"RIGHT\"},\"type\":\"ConnectorPlacement.EquallySpacedRectSide\",\"uuid\":\"5e25e59b-8f8b-4773-b6d9-951d4129523a\"},{\"content\":{\"connectorIds\":[],\"side\":\"TOP\"},\"type\":\"ConnectorPlacement.EquallySpacedRectSide\",\"uuid\":\"bae24e3d-e286-4bf4-a21b-122b1e5bc09f\"},{\"content\":{\"connectorIds\":[\"Out1\"],\"side\":\"BOTTOM\"},\"type\":\"ConnectorPlacement.EquallySpacedRectSide\",\"uuid\":\"0ce66b8b-3f3a-4f1a-9606-df56b31d9b3c\"}]},\"type\":\"ConnectorPlacement.EquallySpacedConnector\",\"uuid\":\"f87c39b6-c8d4-4afb-9096-6dab01ec5afa\"}],\"packageUris\":[\"http://schema.mathworks.com/mf0/Connector/R2020b\"],\"version\":\"1.0\"}"
  Mechanical Rotational Reference1 : fl_lib/Mechanical/Rotational Elements/Mechanical Rotational Reference
  PS-Simulink Converter : nesl_utility/PS-Simulink Converter  PhysicalDomain=network_engine_domain  SubClassName=ps_output  LeftPortType=input  RightPortType=output  PseudoPeriodic=off  Frequencies=[]  VectorFormat=1-D array  Unit=inherit  AffineConversion=off
  Pressure Relief Valve1 : sh_lib/Valves/Pressure Control Valves/Pressure Relief Valve  valve_area_spec=1  p_diff_TLU=[30.15e5 : 15e3 : 31.35e5] Pa  area_TLU=[1 : 1 : 9] .* 1e-5 m^2  area_max=(3.557e-4) m^2  pres_set=PressureValveMax psi  reg_range=ValvePreRange psi  C_d=0.7  A_leak=1e-12 m^2  lam_spec=1  B_lam=0.999  Re_cr=12  dynamic=0  tau=0.1 s  area_init=1e-12 m^2
      settings: InternalSimscapePortConfiguration="{\"Bottom\":[],\"Left\":[{\"id\":\"A\",\"label\":\"A\",\"type\":\"foundation.hydraulic.hydraulic\"}],\"Right\":[{\"id\":\"B\",\"label\":\"B\",\"type\":\"foundation.hydraulic.hydraulic\"}],\"Top\":[]}"
  PressureSensor : Subsystem
  Simulink-PS Converter : nesl_utility/Simulink-PS Converter  PhysicalDomain=network_engine_domain  SubClassName=ps_input  LeftPortType=input  RightPortType=output  PseudoPeriodic=off  Frequencies=[]  NoiseDistribution=none  NoiseParameters=[]  Unit=1  AffineConversion=off  FilteringAndDerivatives=provide  SimscapeFilterOrder=1  InputFilterTimeConstant=0.001  UdotUserProvided=0
  Simulink-PS Converter1 : nesl_utility/Simulink-PS Converter  PhysicalDomain=network_engine_domain  SubClassName=ps_input  LeftPortType=input  RightPortType=output  PseudoPeriodic=off  Frequencies=[]  NoiseDistribution=none  NoiseParameters=[]  Unit=1  AffineConversion=off  FilteringAndDerivatives=provide  SimscapeFilterOrder=1  InputFilterTimeConstant=0.001  UdotUserProvided=0
  Simulink-PS Converter2 : nesl_utility/Simulink-PS Converter  PhysicalDomain=network_engine_domain  SubClassName=ps_input  LeftPortType=input  RightPortType=output  PseudoPeriodic=off  Frequencies=[]  NoiseDistribution=none  NoiseParameters=[]  Unit=1  AffineConversion=off  FilteringAndDerivatives=provide  SimscapeFilterOrder=1  InputFilterTimeConstant=0.001  UdotUserProvided=0
  Solver Configuration : nesl_utility/Solver Configuration  PhysicalDomain=network_engine_domain  SubClassName=solver  LeftPortType=input  RightPortType=generic  Tones=[]  Harmonics=[]  SimulateNoise=off  Profile=off  UseLocalSampling=off  EnableSwitchedLinearOptims=on  FrequencyDomain=off  UseCCode=off  RelTol=0.001  AbsTol=1e-06  MinStep=1e-09  ToWorkspace=off  RevertToSquareIcSolve=off  NumHomotopyIterations=100  PhasorMode=off  PhasorModeNumHarmonics=1  ConsistencySolver=NEWTON_FTOL  IndexReductionMethod=DerivativeReplacement  DoDC=off  ResidualTolerance=1e-09  ConsistencyTolSource=GLOBAL  ConsistencyAbsTol=0.001  ConsistencyRelTol=0.001  ConsistencyTolFactor=0.001  UseLocalSolver=on  LocalSolverChoice=NE_BACKWARD_EULER_ADVANCER  ResolveIndetEquations=on  FunctionEvalNumThread=1  LocalSolverSampleTime=Ts  DoFixedCost=on  MaxNonlinIter=3  MaxModeIter=2  ComputeImpulses=off  ImpulseIterations=2  LinearAlgebra=auto  LinearAlgebraNumThread=0  EquationFormulation=NE_TIME_EF  DelaysMemoryBudget=1024  AutomaticFiltering=on  FilteringTimeConstant=0.001  PartitionStorageMethod=AS_NEEDED  PartitionMemoryBudget=1024  PartitionMethod=ROBUST  MultibodyUseLocalSolver=off  MultibodyLocalSolverChoice=ODE1  MultibodyLocalSolverSampleTime=0.001
  Spring-Loaded Accumulator : sh_lib/Accumulators/Spring-Loaded Accumulator  capacity=AccVol m^3  pr_preload=Acc_PC psi  pr_max=Acc_MaxP psi  stiff_coeff=1e10 Pa/m^3  penetr_coeff=1e10 Pa*s/m^6  flow_rate_specify=off  flow_rate_priority=None  flow_rate=5e-3 m^3/s  flow_rate_nominal_specify=off  flow_rate_nominal_value=1  flow_rate_nominal_unit=m^3/s  fluid_volume_specify=on  fluid_volume_priority=None  fluid_volume=5e-6 m^3  fluid_volume_nominal_specify=off  fluid_volume_nominal_value=1  fluid_volume_nominal_unit=m^3  fluid_pressure_specify=off  fluid_pressure_priority=None  fluid_pressure=1.01325e5 Pa  fluid_pressure_nominal_specify=off  fluid_pressure_nominal_value=1  fluid_pressure_nominal_unit=Pa
      settings: InternalSimscapePortConfiguration="{\"Bottom\":[],\"Left\":[],\"Right\":[{\"id\":\"A\",\"label\":\"A\",\"type\":\"foundation.hydraulic.hydraulic\"}],\"Top\":[]}"
  Subsystem1 : Subsystem
  Subsystem2 : Subsystem
  Subsystem3 : Subsystem
      settings: PortSchema="{\"entries\":[{\"content\":{\"sides\":[{\"content\":{\"connectorIds\":[\"LConn1\"]},\"type\":\"ConnectorPlacement.EquallySpacedRectSide\",\"uuid\":\"7d5827d5-19d2-449a-bfe5-3899d5f2f234\"},{\"content\":{\"connectorIds\":[\"RConn1\"],\"side\":\"RIGHT\"},\"type\":\"ConnectorPlacement.EquallySpacedRectSide\",\"uuid\":\"27ad7fb5-d235-43aa-a783-09c3ddbf3629\"},{\"content\":{\"connectorIds\":[],\"side\":\"TOP\"},\"type\":\"ConnectorPlacement.EquallySpacedRectSide\",\"uuid\":\"41db419c-7193-454e-a54e-cfb74ab94a84\"},{\"content\":{\"connectorIds\":[\"Out1\",\"Out2\"],\"side\":\"BOTTOM\"},\"type\":\"ConnectorPlacement.EquallySpacedRectSide\",\"uuid\":\"63d69fbc-18e5-4f7b-99db-9fcc8740eddf\"}]},\"type\":\"ConnectorPlacement.EquallySpacedConnector\",\"uuid\":\"1d29a5fa-8394-444f-93a2-8698ce035363\"}],\"packageUris\":[\"http://schema.mathworks.com/mf0/Connector/R2020b\"],\"version\":\"1.0\"}"
  Transfer Fcn : TransferFcn  Commented=on  Denominator=[1/(2*pi*50) 1]
  Variable-Displacement Motor1 : sh_lib/Pumps and Motors/Variable-Displacement Motor  mdl_type=2  stroke_max=0.005 m  D_max=Dm_max cm^3/rev  cntrl_mem_tab=[-.0075, 0, .0075] m  displ_tab=[-Dm_max, 0, Dm_max] cm^3/rev  interp_method=1  extrap_method=1  loss_spec=1  w_nominal=nShaftSpeed rpm  pr_nominal=nPreDrop psi  visc_nominal=18 cSt  dens_nominal=900 kg/m^3  efficiency_vol=EffVolNom  no_load_torque=nTorqueNoLoad N*m  torque_pressure_coeff=(1/((200-50)*1e5))*Dm_max*FactorEff*((1-EffMechMax)*nPreDrop-(1-EffMechMin)*nPreDropMin) N*m/Pa  p_diff_eff_TLU=[100000, 1000000, 2000000] Pa  omega_eff_TLU=[25, 50, 100, 200, 300, 400] rad/s  displacement_eff_TLU=[-30, -19, 19, 30] cm^3/rev  vol_eff_TLU=repmat([.816, .908, .954, .977, .981, .984; .325, .663, .831, .916, .925, .946; .137, .568, .78, .892, .893, .91], 1, 1, 4)  mech_eff_TLU=repmat([.996, .996, .996, .996, .996, .996; .988, .989, .989, .989, .989, .99; .981, .981, .982, .982, .983, .984], 1, 1, 4)  p_diff_loss_TLU=[100000, 1000000, 2000000] Pa  omega_loss_TLU=[25, 50, 100, 200, 300, 400] rad/s  displacement_loss_TLU=[-30, -19, 19, 30] cm^3/rev  vol_loss_TLU=repmat([.0282, .0253, .0241, .0235, .0291, .0325; .2596, .1271, .1017, .0917, .1216, .1142; .7874, .1901, .141, .1211, .1797, .1978] * 1e-3, 1, 1, 4) m^3/s  mech_loss_TLU=repmat([.002, .002, .002, .002, .002, .002; .06, .055, .055, .055, .055, .05; .19, .19, .18, .18, .17, .16], 1, 1, 4) N*m  pressure_threshold=1e5 Pa  omega_threshold=10 rad/s  displacement_threshold=0.0001 cm^3/rev  octant_check=0  pressure_check=0  min_valid_pressure=0 Pa  vol_eff_min=1e-3  vol_eff_max=1  mech_eff_min=1e-3  mech_eff_max=1
      settings: InternalSimscapePortConfiguration="{\"Bottom\":[],\"Left\":[{\"id\":\"A\",\"label\":\"A\",\"type\":\"foundation.hydraulic.hydraulic\"},{\"id\":\"C\",\"label\":\"C\",\"type\":\"input\"},{\"id\":\"B\",\"label\":\"B\",\"type\":\"foundation.hydraulic.hydraulic\"}],\"Right\":[{\"id\":\"S\",\"label\":\"S\",\"type\":\"foundation.mechanical.rotational.rotational\"}],\"Top\":[]}"
  Variable-Displacement Motor3 : sh_lib/Pumps and Motors/Variable-Displacement Motor  mdl_type=2  stroke_max=0.005 m  D_max=Dm_max cm^3/rev  cntrl_mem_tab=[-.0075, 0, .0075] m  displ_tab=[-Dm_max, 0, Dm_max] cm^3/rev  interp_method=1  extrap_method=1  loss_spec=1  w_nominal=nShaftSpeed rpm  pr_nominal=nPreDrop psi  visc_nominal=18 cSt  dens_nominal=900 kg/m^3  efficiency_vol=EffVolNom  no_load_torque=nTorqueNoLoad N*m  torque_pressure_coeff=(1/((200-50)*1e5))*Dm_max*FactorEff*((1-EffMechMax)*nPreDrop-(1-EffMechMin)*nPreDropMin) N*m/Pa  p_diff_eff_TLU=[100000, 1000000, 2000000] Pa  omega_eff_TLU=[25, 50, 100, 200, 300, 400] rad/s  displacement_eff_TLU=[-30, -19, 19, 30] cm^3/rev  vol_eff_TLU=repmat([.816, .908, .954, .977, .981, .984; .325, .663, .831, .916, .925, .946; .137, .568, .78, .892, .893, .91], 1, 1, 4)  mech_eff_TLU=repmat([.996, .996, .996, .996, .996, .996; .988, .989, .989, .989, .989, .99; .981, .981, .982, .982, .983, .984], 1, 1, 4)  p_diff_loss_TLU=[100000, 1000000, 2000000] Pa  omega_loss_TLU=[25, 50, 100, 200, 300, 400] rad/s  displacement_loss_TLU=[-30, -19, 19, 30] cm^3/rev  vol_loss_TLU=repmat([.0282, .0253, .0241, .0235, .0291, .0325; .2596, .1271, .1017, .0917, .1216, .1142; .7874, .1901, .141, .1211, .1797, .1978] * 1e-3, 1, 1, 4) m^3/s  mech_loss_TLU=repmat([.002, .002, .002, .002, .002, .002; .06, .055, .055, .055, .055, .05; .19, .19, .18, .18, .17, .16], 1, 1, 4) N*m  pressure_threshold=1e5 Pa  omega_threshold=10 rad/s  displacement_threshold=0.00001 cm^3/rev  octant_check=0  pressure_check=0  min_valid_pressure=0 Pa  vol_eff_min=1e-3  vol_eff_max=1  mech_eff_min=1e-3  mech_eff_max=1
      settings: InternalSimscapePortConfiguration="{\"Bottom\":[],\"Left\":[{\"id\":\"A\",\"label\":\"A\",\"type\":\"foundation.hydraulic.hydraulic\"},{\"id\":\"C\",\"label\":\"C\",\"type\":\"input\"},{\"id\":\"B\",\"label\":\"B\",\"type\":\"foundation.hydraulic.hydraulic\"}],\"Right\":[{\"id\":\"S\",\"label\":\"S\",\"type\":\"foundation.mechanical.rotational.rotational\"}],\"Top\":[]}"
  SystemOutputs : Outport
  Pressure : Outport  Port=2
  hmOutputShaftTorque : Outport  Port=3
  genShaftSpeed_rpm : Outport  Port=4
  excShaftSpeed_rpm : Outport  Port=5
  excShaftTorque_Nm : Outport  Port=6
  genPumpFlow_lpm : Outport  Port=7
  wires:
  [wShaft] -> Bus Creator/1  "wShaft"
  PressureSensor/1(Pressure) -> Pressure/1, [Pressure]
  Bus Creator/1 -> SystemOutputs/1  "SystemOutputs"
  ControlSignal1/1 -> Subsystem1/1(In1)  "cs1"
  Subsystem1/1(Out1) -> Simulink-PS Converter/1
  Subsystem2/1(Out1) -> Simulink-PS Converter1/1
  ControlSignal2/1 -> Subsystem2/1(1)  "cs2"
  FlowSensor/1(FlowPump1) -> [FlowPump1]
  [FlowPump1] -> Bus Creator/2  "FlowPump1"
  [Pressure] -> Bus Creator/3  "Pressure"
  Subsystem3/1(torque_Nm) -> excShaftTorque_Nm/1, [TorqueShaftInput]
  [TorqueShaftInput] -> Bus Creator/4  "TorqueShaftInput"
  LinearVelInput/1(Output) -> [LinearInput]
  [LinearInput] -> Bus Selector/1
  Bus Selector/2 -> Bus Creator/6  "<LinearSpeedInput>"
  Bus Selector/1 -> Bus Creator/5  "<ForceInput>"
  Bus Selector/3 -> Bus Creator/7  "<LinearPositionInput>"
  Fexc/1 -> LinearVelInput/1(Fexc)
  genSpeedActual_rpm/1 -> [wShaft], Gain/1, genShaftSpeed_rpm/1
  FlowSensor2/1(HMFlow_lpm) -> genPumpFlow_lpm/1
  Subsystem3/2(speed_rpm) -> excShaftSpeed_rpm/1
  Gain/1 -> Simulink-PS Converter2/1
  PS-Simulink Converter/1 -> hmOutputShaftTorque/1
  connections:
  FlowSensor1/LConn1 -- FlowSensor/RConn1 -- Pressure Relief Valve1/LConn1 -- FlowSensor2/LConn1 -- ChargeCircuit/LConn1
  PressureSensor/LConn1 -- FlowSensor/LConn1 -- Variable-Displacement Motor1/LConn1
  Variable-Displacement Motor3/LConn2 -- Simulink-PS Converter1/RConn1
  Simulink-PS Converter/RConn1 -- Variable-Displacement Motor1/LConn2
  Spring-Loaded Accumulator/RConn1 -- FlowSensor1/RConn1
  Variable-Displacement Motor3/LConn1 -- FlowSensor2/RConn1
  Subsystem3/RConn1 -- Variable-Displacement Motor1/RConn1
  LinearVelInput/LConn1 -- Subsystem3/LConn1
  Variable-Displacement Motor1/LConn3 -- Pressure Relief Valve1/RConn1 -- Variable-Displacement Motor3/LConn3 -- Hydraulic Reference1/LConn1 -- ChargeCircuit/RConn1 -- Solver Configuration/RConn1 -- Hydraulic Fluid/RConn1
  Simulink-PS Converter2/RConn1 -- Ideal Angular Velocity Source/RConn1
  Mechanical Rotational Reference1/LConn1 -- Ideal Angular Velocity Source/RConn2
  Ideal Torque Sensor/RConn1 -- Variable-Displacement Motor3/RConn1
  PS-Simulink Converter/LConn1 -- Ideal Torque Sensor/RConn2
  Ideal Angular Velocity Source/LConn1 -- Ideal Torque Sensor/LConn1
